simulink model "Practica_1"  (R2024a)
settings: Solver=VariableStepAuto  StartTime=0.0  StopTime=10.0  RelTol=1e-3
InitFcn:
  | m1 = 0.2;
  | l1 = 0.3;
  | m2 = 0.1;
  | l2 = 0.25;
  | g = 9.81;
settings Model: SnapshotBufferSize=2

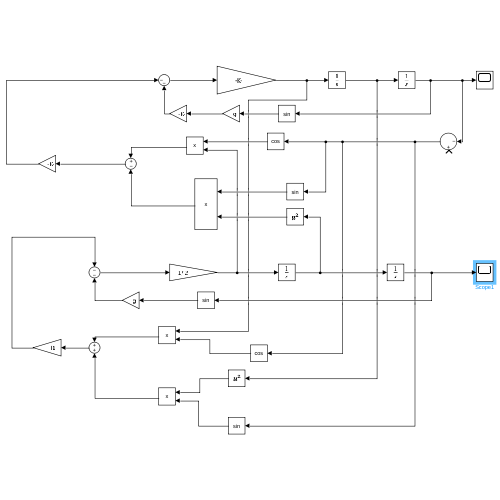
[thumbnail: Simulink's stored preview of the top-level diagram]
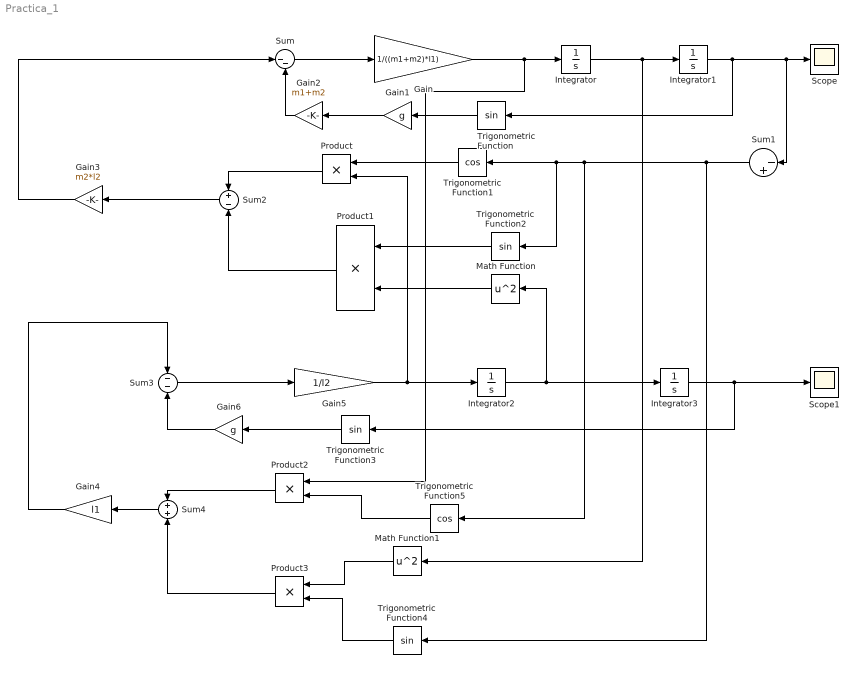
== system Practica_1 ==
  Gain : Gain  Gain=1/((m1+m2)*l1)
  Gain1 : Gain  Gain=g
  Gain2 : Gain  Gain=m1+m2
  Gain3 : Gain  Gain=m2*l2
  Gain4 : Gain  Gain=l1
  Gain5 : Gain  Gain=1/l2
  Gain6 : Gain  Gain=g
  Integrator : Integrator
  Integrator1 : Integrator
  Integrator2 : Integrator
  Integrator3 : Integrator  InitialCondition=(35*pi)/180
  Math Function : Math  Operator=square
  Math Function1 : Math  Operator=square
  Product{,1..3} (4 alike) : Product
  Scope : Scope
  Scope1 : Scope
  Sum : Sum  Inputs=|--
  Sum1 : Sum  Inputs=|-+
  Sum2 : Sum  Inputs=+-
  Sum3 : Sum  Inputs=--
  Sum4 : Sum
  Trigonometric Function{,2..4} (4 alike) : Trigonometry
  Trigonometric Function1 : Trigonometry  Operator=cos
  Trigonometric Function5 : Trigonometry  Operator=cos
  wires:
  Sum/1 -> Gain/1
  Gain/1 -> Product2/1, Integrator/1
  Integrator/1 -> Math Function1/1, Integrator1/1
  Integrator1/1 -> Trigonometric Function/1, Sum1/1, Scope/1
  Gain1/1 -> Gain2/1
  Gain2/1 -> Sum/2
  Trigonometric Function/1 -> Gain1/1
  Gain3/1 -> Sum/1
  Sum2/1 -> Gain3/1
  Product/1 -> Sum2/1
  Product1/1 -> Sum2/2
  Trigonometric Function1/1 -> Product/1
  Trigonometric Function2/1 -> Product1/1
  Math Function/1 -> Product1/2
  Sum1/1 -> Trigonometric Function4/1, Trigonometric Function5/1, Trigonometric Function1/1, Trigonometric Function2/1
  Gain4/1 -> Sum3/1
  Sum3/1 -> Gain5/1
  Gain5/1 -> Product/2, Integrator2/1
  Integrator2/1 -> Math Function/1, Integrator3/1
  Integrator3/1 -> Trigonometric Function3/1, Scope1/1
  Gain6/1 -> Sum3/2
  Trigonometric Function3/1 -> Gain6/1
  Sum4/1 -> Gain4/1
  Product2/1 -> Sum4/1
  Product3/1 -> Sum4/2
  Math Function1/1 -> Product3/1
  Trigonometric Function4/1 -> Product3/2
  Trigonometric Function5/1 -> Product2/2
